simulink model "ReleaseQueue3_Model"  (R2025a)
settings: Solver=VariableStepAuto  StartTime=0.0  StopTime=10.0  RelTol=1e-3
libraries: NSA_DEVS_LOGISTICS x5, NSA_DEVS_SINKS x4, NSA_DEVS_SOURCES x2
settings Model: Creator=peter  LastModifiedBy=peter

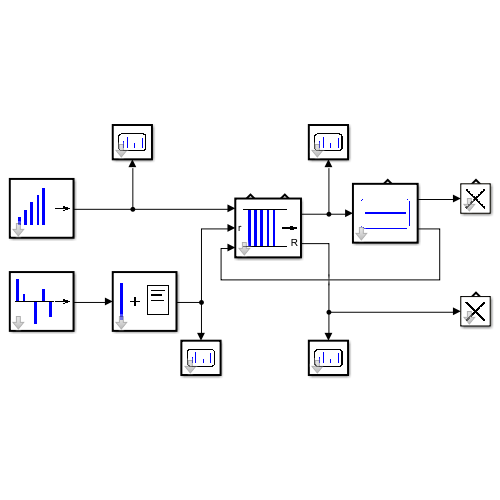
[thumbnail: Simulink's stored preview of the top-level diagram]
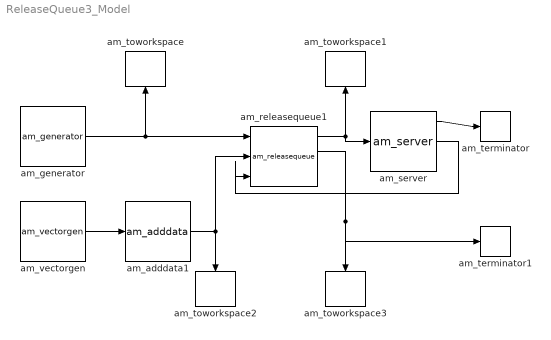
== system ReleaseQueue3_Model ==
  am_adddata1 : NSA_DEVS_LOGISTICS/am_adddata  fields=[]  values=[]  numeric=[]  infield="\"queuePosition_\""  tau=[0,1]  debug=0
      settings: SourceProductName=Logistics
  am_generator : NSA_DEVS_SOURCES/am_generator  tG=3  n0=1  nG=2  tD=[0,2]  debug=0
      settings: SourceProductName=Sources
  am_releasequeue1 : NSA_DEVS_LOGISTICS/am_releasequeue  useSingleElementBatch=false  tD=[0,2]  tau=[0,1]  debug=1
      settings: SourceProductName=Logistics
  am_server : NSA_DEVS_LOGISTICS/am_server  tS=5  tsField="\"\""  tau=[0,1]  debug=0
      settings: SourceProductName=Logistics
  am_terminator : NSA_DEVS_LOGISTICS/am_terminator  tau=[0,1]  debug=0
      settings: SourceProductName=Logistics
  am_terminator1 : NSA_DEVS_LOGISTICS/am_terminator  tau=[0,1]  debug=0
      settings: SourceProductName=Logistics
  am_toworkspace : NSA_DEVS_SINKS/am_toworkspace  varname="\"in\""  t0=0  format="\"vector\""  tau=[0,5]  debug=0
      settings: SourceProductName=Sinks
  am_toworkspace1 : NSA_DEVS_SINKS/am_toworkspace  varname="\"out\""  t0=0  format="\"vector\""  tau=[0,5]  debug=0
      settings: SourceProductName=Sinks
  am_toworkspace2 : NSA_DEVS_SINKS/am_toworkspace  varname="\"rel\""  t0=0  format="\"vector\""  tau=[0,5]  debug=0
      settings: SourceProductName=Sinks
  am_toworkspace3 : NSA_DEVS_SINKS/am_toworkspace  varname="\"outR\""  t0=0  format="\"vector\""  tau=[0,5]  debug=0
      settings: SourceProductName=Sinks
  am_vectorgen : NSA_DEVS_SOURCES/am_vectorgen  tvec=[7 100]  yvec=[1 42]  tau=[0,1]  debug=0
      settings: SourceProductName=Sources
  wires:
  am_generator/1 -> am_releasequeue1/1, am_toworkspace/1
  am_server/2 -> am_releasequeue1/3
  am_server/1 -> am_terminator/1
  am_vectorgen/1 -> am_adddata1/1
  am_adddata1/1 -> am_releasequeue1/2, am_toworkspace2/1
  am_releasequeue1/2 -> am_terminator1/1, am_toworkspace3/1
  am_releasequeue1/1 -> am_toworkspace1/1, am_server/1
